simulink model "Overforingsfunksjon_Translatorisk_samlet_PID"  (R2023b)
settings: Solver=VariableStepAuto  StartTime=0.0  StopTime=5  RelTol=1e-16
values from neighbouring files (symbols this model uses):
  D_hiv_fart = [M(3),rho_vann*Cd*A_z*Z_2]    [Overforingsfunksjon_Translasjon.m]
  D_jag = [M(1),rho_vann*Cd*A_x*X_2]    [Overforingsfunksjon_Translasjon.m]
  D_svai = [M(2),rho_vann*Cd*A_y*Y_2]    [Overforingsfunksjon_Translasjon.m]
settings Model: Creator=Anne Brit  LastModifiedBy=anneb
settings DataIOCC: InitialState=0.5

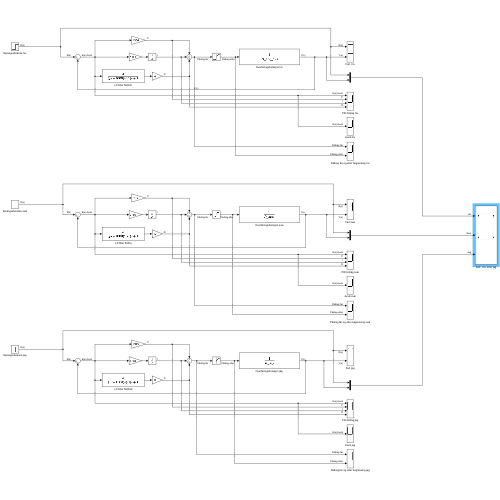
[thumbnail: Simulink's stored preview of the top-level diagram]
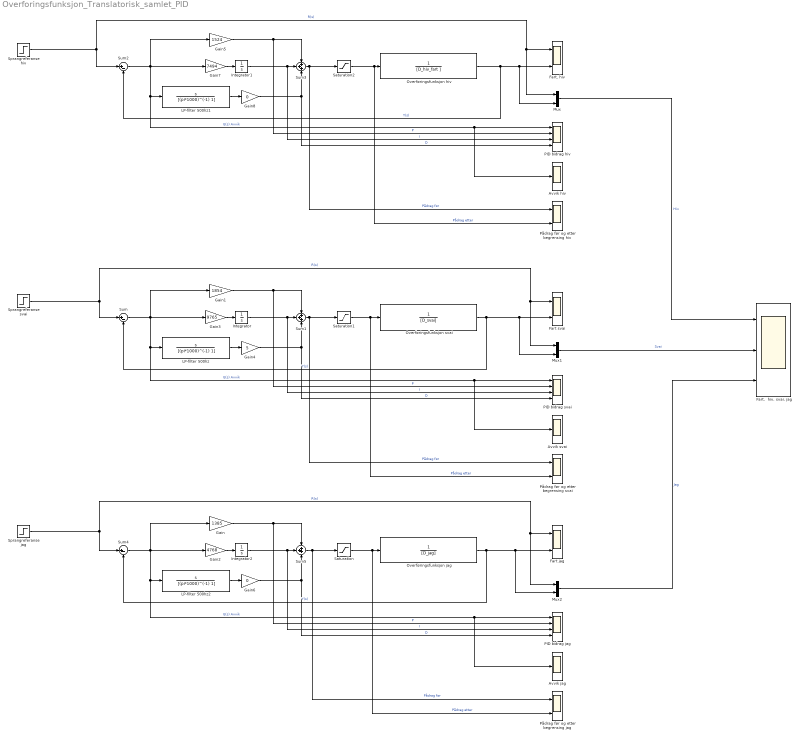
== system Overforingsfunksjon_Translatorisk_samlet_PID ==
  " LP-filter 500hz" : TransferFcn  Numerator=[1 0]  Denominator=[(pi*1000)^(-1) 1]
  " LP-filter 500hz1" : TransferFcn  Numerator=[1 0]  Denominator=[(pi*1000)^(-1) 1]
  " LP-filter 500hz2" : TransferFcn  Numerator=[1 0]  Denominator=[(pi*1000)^(-1) 1]
  Avvik hiv : Scope
  Avvik jag : Scope
  Avvik svai : Scope
  Fart jag : Scope  NumInputPorts=2
  Fart svai : Scope  NumInputPorts=2
  "Fart,  hiv, svai, jag" : Scope  NumInputPorts=3
  "Fart, hiv" : Scope  NumInputPorts=2
  Gain : Gain  Gain=1385
  Gain1 : Gain  Gain=1854
  Gain2 : Gain  Gain=4768
  Gain3 : Gain  Gain=9765
  Gain4 : Gain  Gain=5
  Gain5 : Gain  Gain=1524
  Gain6 : Gain  Gain=0
  Gain7 : Gain  Gain=7494
  Gain8 : Gain  Gain=0
  Integrator : Integrator
  Integrator1 : Integrator
  Integrator2 : Integrator
  Mux : Mux  Inputs=2
  Mux1 : Mux  Inputs=2
  Mux2 : Mux  Inputs=2
  Overføringsfunksjon hiv : TransferFcn  Denominator=[D_hiv_fart ]
  "Overføringsfunksjon jag " : TransferFcn  Denominator=[D_jag]
  Overføringsfunksjon svai : TransferFcn  Denominator=[D_svai]
  PID bidrag hiv : Scope  NumInputPorts=4
  PID bidrag jag : Scope  NumInputPorts=4
  PID bidrag svai : Scope  NumInputPorts=4
  Pådrag før og etter begrensing hiv : Scope  NumInputPorts=2
  Pådrag før og etter begrensing jag : Scope  NumInputPorts=2
  Pådrag før og etter begrensing svai : Scope  NumInputPorts=2
  Saturation : Saturate  UpperLimit=125  LowerLimit=-125
  Saturation1 : Saturate  UpperLimit=65  LowerLimit=-65
  Saturation2 : Saturate  UpperLimit=115  LowerLimit=-145
  Sprangreferanse hiv : Step  After=0.0325  SampleTime=0
  Sprangreferanse jag : Step  After=0.0445  SampleTime=0
  Sprangreferanse svai : Step  After=0.033  SampleTime=0
  Sum : Sum  Inputs=|+-
  Sum1 : Sum  Inputs=+++
  Sum2 : Sum  Inputs=|+-
  Sum3 : Sum  Inputs=+++
  Sum4 : Sum  Inputs=|+-
  Sum5 : Sum  Inputs=+++
  wires:
  Sum5/1 -> Pådrag før og etter begrensing jag/1, Saturation/1  "Pådrag før"
  Integrator2/1 -> PID bidrag jag/3, Sum5/2  "I"
  Sprangreferanse jag/1 -> Sum4/1, Mux2/1, Fart jag/1  "R(s)"
  Sum4/1 -> PID bidrag jag/1, Avvik jag/1, " LP-filter 500hz2"/1, Gain2/1, Gain/1  "E(s) Avvik"
  Saturation/1 -> Pådrag før og etter begrensing jag/2, "Overføringsfunksjon jag "/1  "Pådrag etter"
  "Overføringsfunksjon jag "/1 -> Sum4/2, Mux2/2, Fart jag/2  "Y(s)"
  Gain2/1 -> Integrator2/1
  Gain6/1 -> Sum5/3, PID bidrag jag/4  "D"
  Gain/1 -> Sum5/1, PID bidrag jag/2  "P"
  " LP-filter 500hz2"/1 -> Gain6/1
  Sum1/1 -> Pådrag før og etter begrensing svai/1, Saturation1/1  "Pådrag før"
  Gain3/1 -> Integrator/1
  " LP-filter 500hz"/1 -> Gain4/1
  Gain4/1 -> Sum1/3, PID bidrag svai/4  "D"
  Integrator/1 -> PID bidrag svai/3, Sum1/2  "I"
  Sprangreferanse svai/1 -> Mux1/1, Fart svai/1, Sum/1  "R(s)"
  Saturation1/1 -> Pådrag før og etter begrensing svai/2, Overføringsfunksjon svai/1  "Pådrag etter"
  Gain1/1 -> Sum1/1, PID bidrag svai/2  "P"
  Overføringsfunksjon svai/1 -> Sum/2, Mux1/2, Fart svai/2  "Y(s)"
  Sum/1 -> " LP-filter 500hz"/1, PID bidrag svai/1, Avvik svai/1, Gain3/1, Gain1/1  "E(s) Avvik"
  Saturation2/1 -> Pådrag før og etter begrensing hiv/2, Overføringsfunksjon hiv/1  "Pådrag etter"
  Gain7/1 -> Integrator1/1
  " LP-filter 500hz1"/1 -> Gain8/1
  Integrator1/1 -> PID bidrag hiv/3, Sum3/2  "I"
  Sum3/1 -> Pådrag før og etter begrensing hiv/1, Saturation2/1  "Pådrag før"
  Gain8/1 -> Sum3/3, PID bidrag hiv/4  "D"
  Sprangreferanse hiv/1 -> Sum2/1, Mux/1, "Fart, hiv"/1  "R(s)"
  Sum2/1 -> PID bidrag hiv/1, Avvik hiv/1, " LP-filter 500hz1"/1, Gain7/1, Gain5/1  "E(s) Avvik"
  Overføringsfunksjon hiv/1 -> Sum2/2, Mux/2, "Fart, hiv"/2  "Y(s)"
  Gain5/1 -> Sum3/1, PID bidrag hiv/2  "P"
  Mux/1 -> "Fart,  hiv, svai, jag"/1  "Hiv"
  Mux1/1 -> "Fart,  hiv, svai, jag"/2  "Svai"
  Mux2/1 -> "Fart,  hiv, svai, jag"/3  "Jag"
